simulink model "z1_1"  (R2016b)
settings: Solver=VariableStepAuto  StartTime=0.0  StopTime=10.0  RelTol=1e-3
settings Model: Creator=E7440  LastModifiedBy=E7440

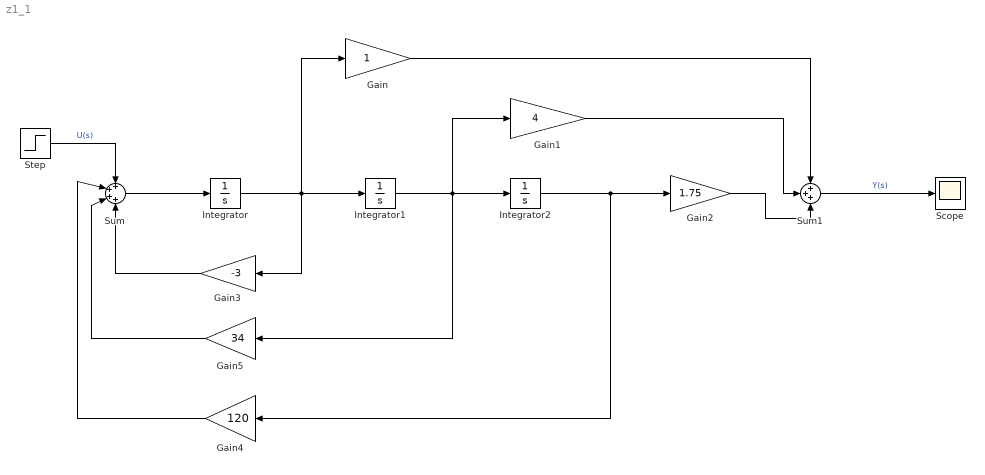
== system z1_1 ==
  Gain : Gain
  Gain1 : Gain  Gain=4
  Gain2 : Gain  Gain=1.75
  Gain3 : Gain  Gain=-3
  Gain4 : Gain  Gain=120
  Gain5 : Gain  Gain=34
  Integrator : Integrator
  Integrator1 : Integrator
  Integrator2 : Integrator
  Scope : Scope
  Step : Step  SampleTime=0
  Sum : Sum  Inputs=++++
  Sum1 : Sum  Inputs=+++
  wires:
  Step/1 -> Sum/1  "U(s)"
  Sum/1 -> Integrator/1
  Gain2/1 -> Sum1/3
  Gain1/1 -> Sum1/2
  Gain/1 -> Sum1/1
  Integrator2/1 -> Gain4/1, Gain2/1
  Integrator/1 -> Integrator1/1, Gain3/1, Gain/1
  Gain3/1 -> Sum/4
  Integrator1/1 -> Integrator2/1, Gain5/1, Gain1/1
  Gain4/1 -> Sum/2
  Gain5/1 -> Sum/3
  Sum1/1 -> Scope/1  "Y(s)"
